simulink subsystem "thermal_controller"  (R2023a)
settings: Solver=VariableStepAuto  StartTime=0.0  StopTime=10.0  RelTol=1e-3
libraries: eeGeneralControl x4, simulink x3, slpidlib x2
settings Model: Creator=daniel.harlander  LastModifiedBy=stefan.notter
settings OptimizationCC: ReuseModelBlockBuffer=off

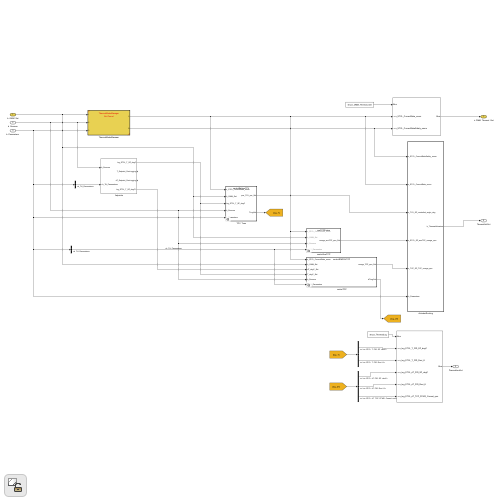
[thumbnail: Simulink's stored preview of the top-level diagram]
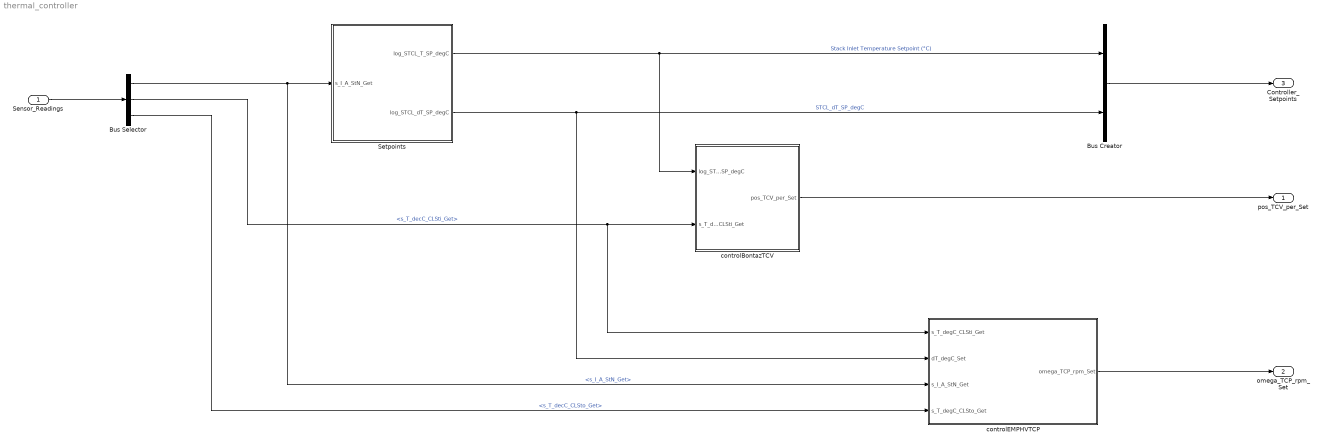
== system thermal_controller ==
  Sensor_Readings : Inport
  Bus Creator : BusCreator  Inputs=2
  Bus Selector : BusSelector  OutputSignals=s_I_A_StN_Get,s_T_decC_CLSti_Get,s_T_decC_CLSto_Get
  Setpoints : Subsystem
  controlBontazTCV : Subsystem  TreatAsAtomicUnit=on  VariantControl=variantConfig.TCV == VARIANT_TCV.BontazCAN
      settings: RTWFcnNameOpts=Use subsystem name  RTWFileNameOpts=Use subsystem name
  controlEMPHVTCP : Subsystem  TreatAsAtomicUnit=on  VariantControl=variantConfig.TCP == VARIANT_TCP.HVPump
  pos_TCV_per_Set : Outport
  omega_TCP_rpm_Set : Outport  Port=2
  Controller_Setpoints : Outport  Port=3
  wires:
  Setpoints/1(log_STCL_T_SP_degC) -> Bus Creator/1, controlBontazTCV/1(log_STCL_T_SP_degC)  "Stack Inlet Temperature Setpoint (°C)"
  Setpoints/2(log_STCL_dT_SP_degC) -> controlEMPHVTCP/2(dT_degC_Set), Bus Creator/2  "STCL_dT_SP_degC"
  controlEMPHVTCP/1(omega_TCP_rpm_Set) -> omega_TCP_rpm_Set/1
  Sensor_Readings/1 -> Bus Selector/1
  Bus Selector/1 -> Setpoints/1(s_I_A_StN_Get), controlEMPHVTCP/3(s_I_A_StN_Get)  "<s_I_A_StN_Get>"
  Bus Selector/2 -> controlBontazTCV/2(s_T_decC_CLSti_Get), controlEMPHVTCP/1(s_T_degC_CLSti_Get)  "<s_T_decC_CLSti_Get>"
  Bus Selector/3 -> controlEMPHVTCP/4(s_T_degC_CLSto_Get)  "<s_T_decC_CLSto_Get>"
  controlBontazTCV/1(pos_TCV_per_Set) -> pos_TCV_per_Set/1
  Bus Creator/1 -> Controller_Setpoints/1

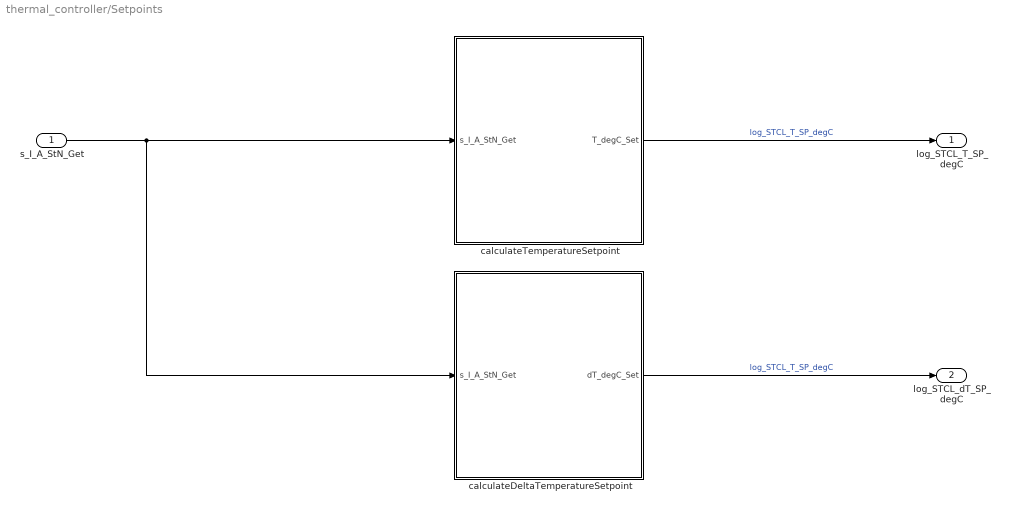
== system thermal_controller/Setpoints ==
  s_I_A_StN_Get : Inport
  calculateDeltaTemperatureSetpoint : Subsystem  TreatAsAtomicUnit=on
      settings: RTWSystemCode=Nonreusable function  RTWFcnNameOpts=Use subsystem name  RTWFileNameOpts=Use subsystem name
  calculateTemperatureSetpoint : Subsystem  TreatAsAtomicUnit=on
      settings: RTWSystemCode=Nonreusable function  RTWFcnNameOpts=Use subsystem name  RTWFileNameOpts=Use subsystem name
  log_STCL_T_SP_degC : Outport
  log_STCL_dT_SP_degC : Outport  Port=2
  wires:
  calculateTemperatureSetpoint/1(T_degC_Set) -> log_STCL_T_SP_degC/1  "log_STCL_T_SP_degC"
  calculateDeltaTemperatureSetpoint/1(dT_degC_Set) -> log_STCL_dT_SP_degC/1  "log_STCL_T_SP_degC"
  s_I_A_StN_Get/1 -> calculateDeltaTemperatureSetpoint/1(s_I_A_StN_Get), calculateTemperatureSetpoint/1(s_I_A_StN_Get)

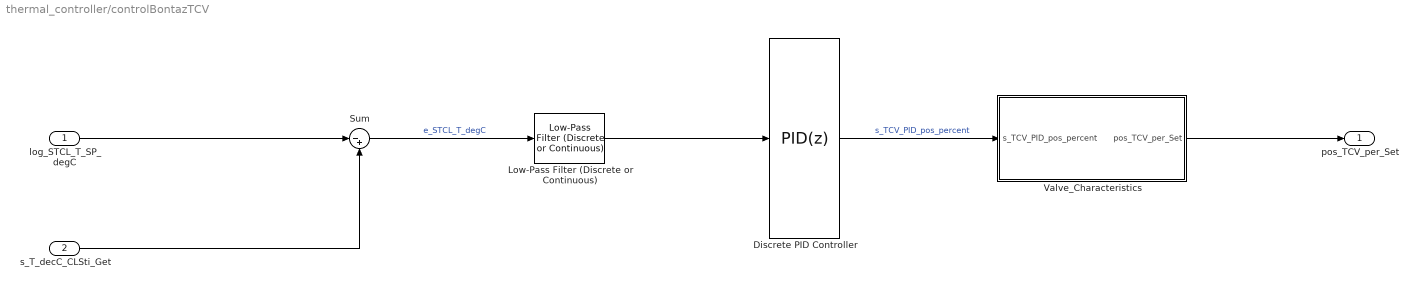
== system thermal_controller/controlBontazTCV ==
  log_STCL_T_SP_degC : Inport
  s_T_decC_CLSti_Get : Inport  Port=2
  Discrete PID Controller : slpidlib/PID Controller  Controller=PID  Form=Parallel  TimeDomain=Discrete-time  UseExternalTs=off  SampleTime=-1  IntegratorMethod=Forward Euler  FilterMethod=Forward Euler  ControllerParametersSource=internal  P=2  I=0.75  UseKiTs=off  D=0  N=100  UseFilter=off  TunerSelectOption=Transfer Function Based (PID Tuner App)  InitialConditionSource=internal  InitialConditionForIntegrator=0  InitialConditionForFilter=0  DifferentiatorICPrevScaledInput=0  ExternalReset=none  TrackingMode=off  Kt=1  LimitOutput=on  SatLimitsSource=internal  UpperSaturationLimit=100  LowerSaturationLimit=0  LinearizeAsGain=on  AntiWindupMode=clamping  Kb=1  LimitIntegrator=off  UpperIntegratorSaturationLimit=inf  LowerIntegratorSaturationLimit=-inf  POutMin=[]  POutMax=[]  IOutMin=[]  IOutMax=[]  DOutMin=[]  DOutMax=[]  NOutMin=[]  NOutMax=[]  SumOutMin=[]  SumOutMax=[]  SaturationOutMin=[]  SaturationOutMax=[]  PParamMin=[]  PParamMax=[]  IParamMin=[]  IParamMax=[]  DParamMin=[]  DParamMax=[]  NParamMin=[]  NParamMax=[]  KbParamMin=[]  KbParamMax=[]  KtParamMin=[]  KtParamMax=[]  KbOutMin=[]  KbOutMax=[]  KtOutMin=[]  KtOutMax=[]  IntegratorOutMin=[]  IntegratorOutMax=[]  FilterOutMin=[]  FilterOutMax=[]  SumI1OutMin=[]  SumI1OutMax=[]  SumI2OutMin=[]  SumI2OutMax=[]  SumI3OutMin=[]  SumI3OutMax=[]  SumI4OutMin=[]  SumI4OutMax=[]  SumDOutMin=[]  SumDOutMax=[]  DifferentiatorOutMin=[]  DifferentiatorOutMax=[]  FilterDiffOutCoefMin=[]  FilterDiffOutCoefMax=[]  ReciprocalOutMin=[]  ReciprocalOutMax=[]  SumDenOutMin=[]  SumDenOutMax=[]  SumNumOutMin=[]  SumNumOutMax=[]  DivideOutMin=[]  DivideOutMax=[]  UdiffTsProdOutMin=[]  UdiffTsProdOutMax=[]  NTsProdOutMin=[]  NTsProdOutMax=[]  UintegralTsProdOutMin=[]  UintegralTsProdOutMax=[]  UngainTsProdOutMin=[]  UngainTsProdOutMax=[]  ClampingZeroOutDataTypeStr=Inherit: Inherit via back propagation  ClampingZeroOutMin=[]  ClampingZeroOutMax=[]  FilterDenConstantOutDataTypeStr=Inherit: Inherit via back propagation  FilterDenConstantOutMin=[]  FilterDenConstantOutMax=[]  PCopyOutDataTypeStr=Inherit: Inherit via back propagation  PCopyOutMin=[]  PCopyOutMax=[]  NCopyOutDataTypeStr=Inherit: Inherit via back propagation  NCopyOutMin=[]  NCopyOutMax=[]  IntegratorContinuousStateAttributes=''  IntegratorStateMustResolveToSignalObject=off  IntegratorRTWStateStorageClass=Auto  FilterContinuousStateAttributes=''  FilterStateMustResolveToSignalObject=off  FilterRTWStateStorageClass=Auto  ParallelPVariant=InternalParameters  IdealPVariant=Disabled  IVariant=InternalParameters  DVariant=InternalParameters  IntegratorVariant=Discrete  SatVariant=Enabled  AWVariant=DiscClampingParallel  PCopyVariant=Disabled  TRVariant=Disabled  FdbkBlocksVariant=Forward  IdealPFdbkVariant=Disabled  SatFdbkVariant=Disabled  DerivativeFilterVariant=Differentiator  NVariant=Passthrough  NCopyVariant=Disabled_SignalSpec  FilterICVariant=InternalICsDifferentiator  IntegratorICVariant=InternalICs  ExternalResetVariant=Disabled  TRSumVariant=Passthrough  SumFdbkVariant=Disabled  SumVariant=Sum_PID  TsampFilterVariant=InternalTs  TsampNgainVariant=Passthrough  TsampIntegralVariant=Disabled_SignalSpec  ExternalSaturationOutDataTypeStr=Inherit: Same as second input
      settings: LibrarySourceBlock=simulink/Discrete/Discrete PID Controller
  Low-Pass Filter (Discrete or Continuous) : eeGeneralControl/Low-Pass Filter (Discrete or Continuous)  K=1  T=1  B=inf  A=-inf  init_option=Inherited from block input  x0=0  Ts=-1
  Sum : Sum  Inputs=|-+
  Valve_Characteristics : Subsystem
  pos_TCV_per_Set : Outport
  wires:
  s_T_decC_CLSti_Get/1 -> Sum/2
  log_STCL_T_SP_degC/1 -> Sum/1
  Sum/1 -> Low-Pass Filter (Discrete or Continuous)/1  "e_STCL_T_degC"
  Low-Pass Filter (Discrete or Continuous)/1 -> Discrete PID Controller/1
  Discrete PID Controller/1 -> Valve_Characteristics/1(s_TCV_PID_pos_percent)  "s_TCV_PID_pos_percent"
  Valve_Characteristics/1(pos_TCV_per_Set) -> pos_TCV_per_Set/1

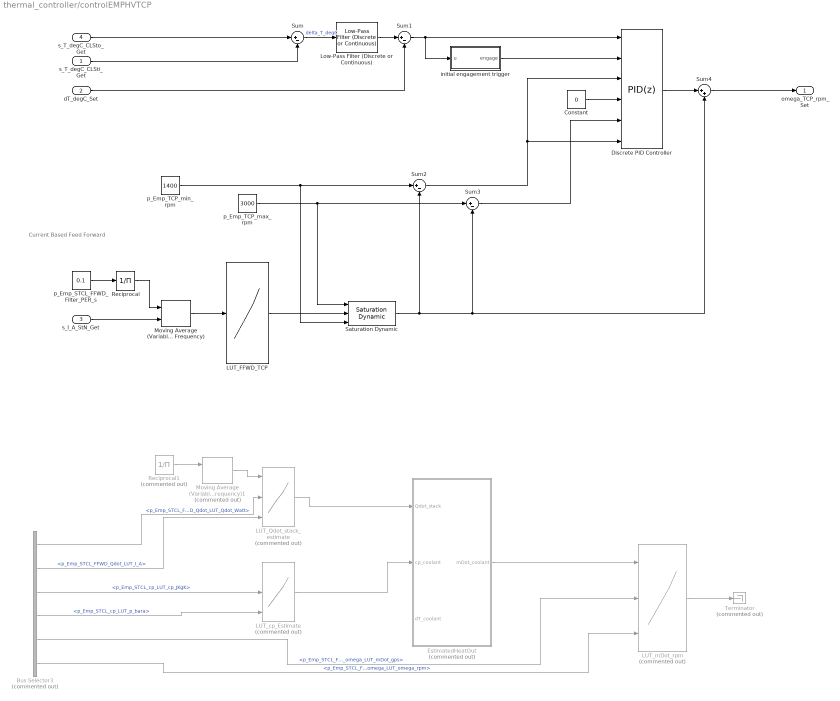
== system thermal_controller/controlEMPHVTCP ==
  note: Current Based Feed Forward
  s_T_degC_CLSti_Get : Inport
  dT_degC_Set : Inport  Port=2
  s_I_A_StN_Get : Inport  Port=3
  s_T_degC_CLSto_Get : Inport  Port=4
  Bus Selector3 : BusSelector  Commented=on  OutputSignals=b_STCL_Parameters.p_Emp_STCL_FFWD_Qdot_LUT_Qdot_Watt,b_STCL_Parameters.p_Emp_STCL_FFWD_Qdot_LUT_I_A,b_STCL_Parameters.p_Emp_STCL_cp_LUT_cp_JKgK,b_STCL_Parameters.p_Emp_STCL_cp_LUT_p_bara,b_STCL_Parameters.p_Emp_STCL_FFWD_omega_LUT_mDot_gps,b_STCL_Parameters.p_Emp_STCL_FFWD_omega_LUT_omega_rpm
  Constant : Constant  Value=0  OutDataTypeStr=single
  Discrete PID Controller : slpidlib/PID Controller  Controller=PID  Form=Parallel  TimeDomain=Discrete-time  UseExternalTs=off  SampleTime=-1  IntegratorMethod=Forward Euler  FilterMethod=Forward Euler  ControllerParametersSource=internal  P=50  I=5  UseKiTs=off  D=0  N=100  UseFilter=off  TunerSelectOption=Transfer Function Based (PID Tuner App)  InitialConditionSource=external  InitialConditionForIntegrator=0  InitialConditionForFilter=0  DifferentiatorICPrevScaledInput=0  ExternalReset=rising  TrackingMode=off  Kt=1  LimitOutput=on  SatLimitsSource=external  UpperSaturationLimit=inf  LowerSaturationLimit=-inf  LinearizeAsGain=on  AntiWindupMode=clamping  Kb=1  LimitIntegrator=off  UpperIntegratorSaturationLimit=inf  LowerIntegratorSaturationLimit=-inf  POutMin=[]  POutMax=[]  IOutMin=[]  IOutMax=[]  DOutMin=[]  DOutMax=[]  NOutMin=[]  NOutMax=[]  SumOutMin=[]  SumOutMax=[]  SaturationOutMin=[]  SaturationOutMax=[]  PParamMin=[]  PParamMax=[]  IParamMin=[]  IParamMax=[]  DParamMin=[]  DParamMax=[]  NParamMin=[]  NParamMax=[]  KbParamMin=[]  KbParamMax=[]  KtParamMin=[]  KtParamMax=[]  KbOutMin=[]  KbOutMax=[]  KtOutMin=[]  KtOutMax=[]  IntegratorOutMin=[]  IntegratorOutMax=[]  FilterOutMin=[]  FilterOutMax=[]  SumI1OutMin=[]  SumI1OutMax=[]  SumI2OutMin=[]  SumI2OutMax=[]  SumI3OutMin=[]  SumI3OutMax=[]  SumI4OutMin=[]  SumI4OutMax=[]  SumDOutMin=[]  SumDOutMax=[]  DifferentiatorOutMin=[]  DifferentiatorOutMax=[]  FilterDiffOutCoefMin=[]  FilterDiffOutCoefMax=[]  ReciprocalOutMin=[]  ReciprocalOutMax=[]  SumDenOutMin=[]  SumDenOutMax=[]  SumNumOutMin=[]  SumNumOutMax=[]  DivideOutMin=[]  DivideOutMax=[]  UdiffTsProdOutMin=[]  UdiffTsProdOutMax=[]  NTsProdOutMin=[]  NTsProdOutMax=[]  UintegralTsProdOutMin=[]  UintegralTsProdOutMax=[]  UngainTsProdOutMin=[]  UngainTsProdOutMax=[]  ClampingZeroOutDataTypeStr=Inherit: Inherit via back propagation  ClampingZeroOutMin=[]  ClampingZeroOutMax=[]  FilterDenConstantOutDataTypeStr=Inherit: Inherit via back propagation  FilterDenConstantOutMin=[]  FilterDenConstantOutMax=[]  PCopyOutDataTypeStr=Inherit: Inherit via back propagation  PCopyOutMin=[]  PCopyOutMax=[]  NCopyOutDataTypeStr=Inherit: Inherit via back propagation  NCopyOutMin=[]  NCopyOutMax=[]  IntegratorContinuousStateAttributes=''  IntegratorStateMustResolveToSignalObject=off  IntegratorRTWStateStorageClass=Auto  FilterContinuousStateAttributes=''  FilterStateMustResolveToSignalObject=off  FilterRTWStateStorageClass=Auto  ParallelPVariant=InternalParameters  IdealPVariant=Disabled  IVariant=InternalParameters  DVariant=InternalParameters  IntegratorVariant=Discrete  SatVariant=External  AWVariant=DiscClampingParallel  PCopyVariant=Disabled  TRVariant=Disabled  FdbkBlocksVariant=Forward  IdealPFdbkVariant=Disabled  SatFdbkVariant=Disabled  DerivativeFilterVariant=Differentiator  NVariant=Passthrough  NCopyVariant=Disabled_SignalSpec  FilterICVariant=ExternalICs  IntegratorICVariant=ExternalICs  ExternalResetVariant=ExternalReset  TRSumVariant=Passthrough  SumFdbkVariant=Disabled  SumVariant=Sum_PID  TsampFilterVariant=InternalTs  TsampNgainVariant=Passthrough  TsampIntegralVariant=Disabled_SignalSpec  ExternalSaturationOutDataTypeStr=Inherit: Same as second input
      settings: LibrarySourceBlock=simulink/Discrete/Discrete PID Controller
  EstimatedHeatOut : MATLAB Function  Commented=on  TreatAsAtomicUnit=on
  LUT_FFWD_TCP : Lookup_n-D  NumberOfTableDimensions=1  BreakpointsForDimension1="[   0,  100,  199,  200,  250,  300,  350,  399,  400,  420,  450,  480,  500,  600]"  Table=[1400, 1400, 1600, 1800, 2200, 2600, 2800, 2900, 2900, 2900, 2900, 2900, 2900, 2900]  ExtrapMethod=Clip  UseLastTableValue=on  InternalRulePriority=Speed  RndMeth=Simplest
  LUT_Qdot_stack_estimate : Lookup_n-D  Commented=on  NumberOfTableDimensions=1  BreakpointsForDimension1Source=Input port  BreakpointsForDimension1=[-5:5]  TableSource=Input port  Table=tanh([-5:5])  ExtrapMethod=Clip  UseLastTableValue=on  InternalRulePriority=Speed  RndMeth=Simplest
      settings: InputPortMap=u0,p221,p5
  LUT_cp_Estimate : Lookup_n-D  Commented=on  NumberOfTableDimensions=1  BreakpointsForDimension1Source=Input port  BreakpointsForDimension1=[-5:5]  TableSource=Input port  Table=tanh([-5:5])  ExtrapMethod=Clip  UseLastTableValue=on  InternalRulePriority=Speed  RndMeth=Simplest
      settings: InputPortMap=u0,p221,p5
  LUT_mDot_rpm : Lookup_n-D  Commented=on  NumberOfTableDimensions=1  BreakpointsForDimension1Source=Input port  BreakpointsForDimension1=[-5:5]  TableSource=Input port  Table=tanh([-5:5])  ExtrapMethod=Clip  UseLastTableValue=on  InternalRulePriority=Speed  RndMeth=Simplest
      settings: InputPortMap=u0,p221,p5
  Low-Pass Filter (Discrete or Continuous) : eeGeneralControl/Low-Pass Filter (Discrete or Continuous)  K=1  T=1  B=inf  A=-inf  init_option=Inherited from block input  x0=0  Ts=-1
  Moving Average (Variable Frequency) : eeGeneralControl/Moving Average (Variable Frequency)  VariantControl=Variant1  LabelModeActiveChoice=Discrete  f0=100  fmin=0.1  x0=0  BufferSize=8192  Ts=-1
      settings: LibrarySourceBlock=|
      | ee_sl_lib/General Control/Moving Average
      | (Variable Frequency)
  Moving Average (Variable Frequency)1 : eeGeneralControl/Moving Average (Variable Frequency)  Commented=on  VariantControl=Variant1  LabelModeActiveChoice=Discrete  f0=100  fmin=0.1  x0=0  BufferSize=8192  Ts=-1
      settings: LibrarySourceBlock=|
      | ee_sl_lib/General Control/Moving Average
      | (Variable Frequency)
  Reciprocal : Product  Inputs=/
  Reciprocal1 : Product  Commented=on  Inputs=/
  Saturation Dynamic : simulink/Discontinuities/Saturation Dynamic  OutMin=[]  OutMax=[]  OutDataTypeStr=Inherit: Same as second input  OutDataType=fixdt(1, 16)  OutScaling=2^-10  DoSatur=off
  Sum{,1..3} (4 alike) : Sum  Inputs=|+-
  Sum4 : Sum  Inputs=|++
  Terminator : Terminator  Commented=on
  initial engagement trigger : Subsystem
  p_Emp_STCL_FFWD_Filter_PER_s : Constant  Value=0.1
  p_Emp_TCP_max_rpm : Constant  Value=3000
  p_Emp_TCP_min_rpm : Constant  Value=1400
  omega_TCP_rpm_Set : Outport
  wires:
  initial engagement trigger/1(engage) -> Discrete PID Controller/2
  LUT_mDot_rpm/1 -> Terminator/1
  Bus Selector3/3 -> LUT_cp_Estimate/2  "<p_Emp_STCL_cp_LUT_cp_JKgK>"
  Bus Selector3/4 -> LUT_cp_Estimate/3  "<p_Emp_STCL_cp_LUT_p_bara>"
  LUT_cp_Estimate/1 -> EstimatedHeatOut/2(cp_coolant)
  Bus Selector3/6 -> LUT_mDot_rpm/3  "<p_Emp_STCL_FFWD_omega_LUT_omega_rpm>"
  Bus Selector3/5 -> LUT_mDot_rpm/2  "<p_Emp_STCL_FFWD_omega_LUT_mDot_gps>"
  Bus Selector3/2 -> LUT_Qdot_stack_estimate/3  "<p_Emp_STCL_FFWD_Qdot_LUT_I_A>"
  Bus Selector3/1 -> LUT_Qdot_stack_estimate/2  "<p_Emp_STCL_FFWD_Qdot_LUT_Qdot_Watt>"
  Reciprocal1/1 -> Moving Average (Variable Frequency)1/1
  Moving Average (Variable Frequency)1/1 -> LUT_Qdot_stack_estimate/1
  EstimatedHeatOut/1(mDot_coolant) -> LUT_mDot_rpm/1
  LUT_Qdot_stack_estimate/1 -> EstimatedHeatOut/1(Qdot_stack)
  Discrete PID Controller/1 -> Sum4/1
  s_T_degC_CLSti_Get/1 -> Sum/2
  p_Emp_TCP_min_rpm/1 -> Saturation Dynamic/3, Sum2/1
  s_T_degC_CLSto_Get/1 -> Sum/1
  Low-Pass Filter (Discrete or Continuous)/1 -> Sum1/1
  Sum1/1 -> Discrete PID Controller/1, initial engagement trigger/1(u)
  p_Emp_TCP_max_rpm/1 -> Sum3/1, Saturation Dynamic/1
  Constant/1 -> Discrete PID Controller/4
  Sum/1 -> Low-Pass Filter (Discrete or Continuous)/1  "delta_T_degC"
  dT_degC_Set/1 -> Sum1/2
  Moving Average (Variable Frequency)/1 -> LUT_FFWD_TCP/1
  s_I_A_StN_Get/1 -> Moving Average (Variable Frequency)/2
  LUT_FFWD_TCP/1 -> Saturation Dynamic/2
  Saturation Dynamic/1 -> Sum4/2, Sum3/2, Sum2/2
  Sum2/1 -> Discrete PID Controller/6, Discrete PID Controller/3
  Sum3/1 -> Discrete PID Controller/5
  Sum4/1 -> omega_TCP_rpm_Set/1
  p_Emp_STCL_FFWD_Filter_PER_s/1 -> Reciprocal/1
  Reciprocal/1 -> Moving Average (Variable Frequency)/1

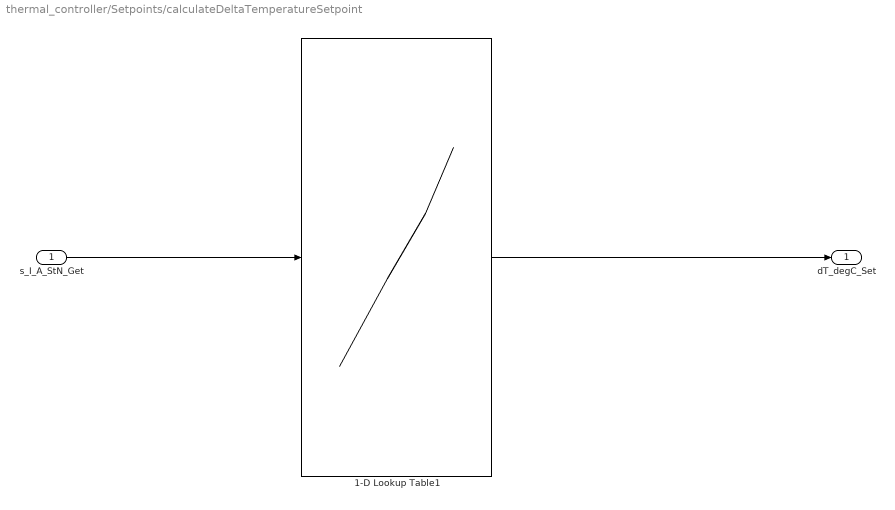
== system thermal_controller/Setpoints/calculateDeltaTemperatureSetpoint ==
  s_I_A_StN_Get : Inport
  1-D Lookup Table1 : Lookup_n-D  NumberOfTableDimensions=1  BreakpointsForDimension1="[0   50   100   150   200   250   300   350   400   425   450   475   500]"  BreakpointsForDimension2Source=Input port  Table="[ 8, 8,    8,    8,     8,    8,    8,    8,     9,   10,   11,   12,   13]"  ExtrapMethod=Clip  InternalRulePriority=Speed  RndMeth=Simplest
  dT_degC_Set : Outport
  wires:
  s_I_A_StN_Get/1 -> 1-D Lookup Table1/1
  1-D Lookup Table1/1 -> dT_degC_Set/1

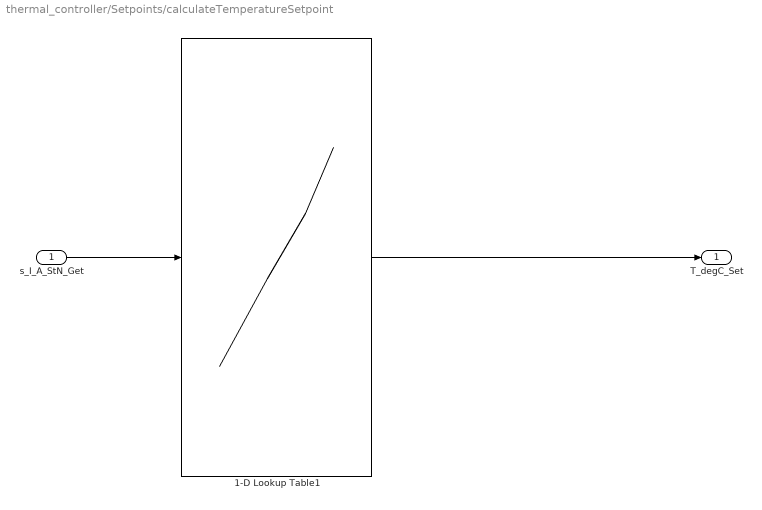
== system thermal_controller/Setpoints/calculateTemperatureSetpoint ==
  s_I_A_StN_Get : Inport
  1-D Lookup Table1 : Lookup_n-D  NumberOfTableDimensions=1  BreakpointsForDimension1="[0   50   100   150   200   250   300   350   400   425   450   475   500]"  BreakpointsForDimension2Source=Input port  Table="[58, 58,   62,   64,   66,   69,   72,  73,   73,   73,   73,   73,   73]"  ExtrapMethod=Clip  InternalRulePriority=Speed  RndMeth=Simplest
  T_degC_Set : Outport
  wires:
  s_I_A_StN_Get/1 -> 1-D Lookup Table1/1
  1-D Lookup Table1/1 -> T_degC_Set/1

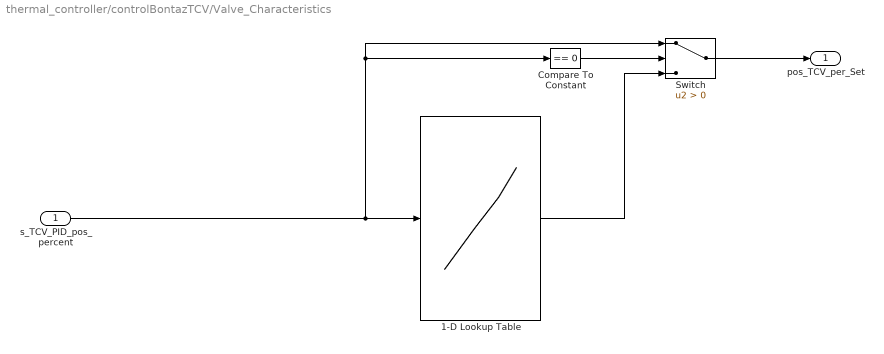
== system thermal_controller/controlBontazTCV/Valve_Characteristics ==
  s_TCV_PID_pos_percent : Inport
  1-D Lookup Table : Lookup_n-D  NumberOfTableDimensions=1  BreakpointsForDimension1="[5  10  70  73 80 100]"  Table="[0  2   91  95 99 100]"  InternalRulePriority=Speed  RndMeth=Simplest
  Compare To Constant : simulink/Logic and Bit Operations/Compare To Constant  relop===  const=0  OutDataTypeStr=boolean
  Switch : Switch  Criteria=u2 > Threshold  SaturateOnIntegerOverflow=off  InputSameDT=off
  pos_TCV_per_Set : Outport
  wires:
  Switch/1 -> pos_TCV_per_Set/1
  1-D Lookup Table/1 -> Switch/3
  Compare To Constant/1 -> Switch/2
  s_TCV_PID_pos_percent/1 -> Compare To Constant/1, Switch/1, 1-D Lookup Table/1

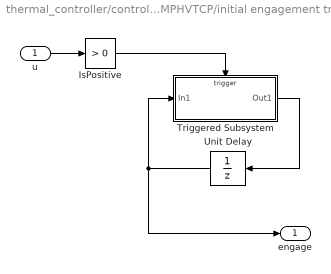
== system thermal_controller/controlEMPHVTCP/initial engagement trigger ==
  u : Inport
  IsPositive : simulink/Logic and Bit Operations/Compare To Zero  relop=>  OutDataTypeStr=boolean
      settings: LibrarySourceBlock=|
      | simulink/Quick Insert/Logic and Bit
      | Operations/IsPositive
  Triggered Subsystem : Subsystem  TreatAsAtomicUnit=on
  Unit Delay : UnitDelay  SampleTime=-1  HasFrameUpgradeWarning=on
  engage : Outport
  wires:
  u/1 -> IsPositive/1
  IsPositive/1 -> Triggered Subsystem/Trigger
  Unit Delay/1 -> engage/1, Triggered Subsystem/1(In1)
  Triggered Subsystem/1(Out1) -> Unit Delay/1

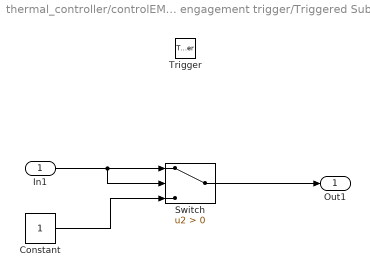
== system thermal_controller/controlEMPHVTCP/initial engagement trigger/Triggered Subsystem ==
  In1 : Inport
  Trigger : TriggerPort  VariantControl=(inherit)
  Constant : Constant  OutDataTypeStr=boolean
  Switch : Switch  Criteria=u2 > Threshold  SaturateOnIntegerOverflow=off  InputSameDT=off
  Out1 : Outport
  wires:
  Constant/1 -> Switch/3
  In1/1 -> Switch/1, Switch/2
  Switch/1 -> Out1/1

== matlab function thermal_controller/controlEMPHVTCP/EstimatedHeatOut ==
  data: Qdot_stack input; mDot_coolant output; cp_coolant input; dT_coolant input
function mDot_coolant = fcn(Qdot_stack, cp_coolant, dT_coolant)

mDot_coolant = Qdot_stack / (cp_coolant * dT_coolant);
